simulink model "gm_parallel_prediction_and_cost_function_6phase"  (R2022a)
settings: Solver=FixedStepDiscrete  StartTime=0.0  StopTime=10.0  RelTol=1e-3
undefined symbols (not defined in the file or in its folder): f_c, L_d, L_q, L_x, L_y, p, psi_pm, R_ph
libraries: hdlmdlgenlib x338
(part 10 of 12)

== system gm_parallel_prediction_and_cost_function_6phase/Prediction_and_cost_function/Subsystem/MATLAB Function14/multiplier9 ==
  In1 : Inport
  In2 : Inport  Port=2
  multiplier9 : Product  Inputs=**  OutDataTypeStr=single  SampleTime=1e-08
  multiplier9_pd1 : Delay  DelayLength=6
  Out1 : Outport
  wires:
  multiplier9_pd1/1 -> Out1/1
  multiplier9/1 -> multiplier9_pd1/1
  In2/1 -> multiplier9/2
  In1/1 -> multiplier9/1

== system gm_parallel_prediction_and_cost_function_6phase/Prediction_and_cost_function/Subsystem/MATLAB Function14/square ==
  In1 : Inport
  In2 : Inport  Port=2
  square : Product  Inputs=**  OutDataTypeStr=single  SampleTime=1e-08
  square_pd1 : Delay  DelayLength=6
  Out1 : Outport
  wires:
  square_pd1/1 -> Out1/1
  square/1 -> square_pd1/1
  In2/1 -> square/2
  In1/1 -> square/1

== system gm_parallel_prediction_and_cost_function_6phase/Prediction_and_cost_function/Subsystem/MATLAB Function14/square1 ==
  In1 : Inport
  In2 : Inport  Port=2
  square1 : Product  Inputs=**  OutDataTypeStr=single  SampleTime=1e-08
  square1_pd1 : Delay  DelayLength=6
  Out1 : Outport
  wires:
  square1_pd1/1 -> Out1/1
  square1/1 -> square1_pd1/1
  In2/1 -> square1/2
  In1/1 -> square1/1

== system gm_parallel_prediction_and_cost_function_6phase/Prediction_and_cost_function/Subsystem/MATLAB Function14/square2 ==
  In1 : Inport
  In2 : Inport  Port=2
  square2 : Product  Inputs=**  OutDataTypeStr=single  SampleTime=1e-08
  square2_pd1 : Delay  DelayLength=6
  Out1 : Outport
  wires:
  square2_pd1/1 -> Out1/1
  square2/1 -> square2_pd1/1
  In2/1 -> square2/2
  In1/1 -> square2/1

== system gm_parallel_prediction_and_cost_function_6phase/Prediction_and_cost_function/Subsystem/MATLAB Function14/square3 ==
  In1 : Inport
  In2 : Inport  Port=2
  square3 : Product  Inputs=**  OutDataTypeStr=single  SampleTime=1e-08
  square3_pd1 : Delay  DelayLength=6
  Out1 : Outport
  wires:
  square3_pd1/1 -> Out1/1
  square3/1 -> square3_pd1/1
  In2/1 -> square3/2
  In1/1 -> square3/1

== system gm_parallel_prediction_and_cost_function_6phase/Prediction_and_cost_function/Subsystem/MATLAB Function14/subtract ==
  In1 : Inport
  In2 : Inport  Port=2
  subtract : Sum  Inputs=+-  OutDataTypeStr=single  SampleTime=1e-08
  subtract_pd1 : Delay  DelayLength=6
  Out1 : Outport
  wires:
  subtract_pd1/1 -> Out1/1
  subtract/1 -> subtract_pd1/1
  In2/1 -> subtract/2
  In1/1 -> subtract/1

== system gm_parallel_prediction_and_cost_function_6phase/Prediction_and_cost_function/Subsystem/MATLAB Function14/subtract1 ==
  In1 : Inport
  In2 : Inport  Port=2
  subtract1 : Sum  Inputs=+-  OutDataTypeStr=single  SampleTime=1e-08
  subtract1_pd1 : Delay  DelayLength=6
  Out1 : Outport
  wires:
  subtract1_pd1/1 -> Out1/1
  subtract1/1 -> subtract1_pd1/1
  In2/1 -> subtract1/2
  In1/1 -> subtract1/1

== system gm_parallel_prediction_and_cost_function_6phase/Prediction_and_cost_function/Subsystem/MATLAB Function14/subtract2 ==
  In1 : Inport
  In2 : Inport  Port=2
  subtract2 : Sum  Inputs=+-  OutDataTypeStr=single  SampleTime=1e-08
  subtract2_pd1 : Delay  DelayLength=6
  Out1 : Outport
  wires:
  subtract2_pd1/1 -> Out1/1
  subtract2/1 -> subtract2_pd1/1
  In2/1 -> subtract2/2
  In1/1 -> subtract2/1

== system gm_parallel_prediction_and_cost_function_6phase/Prediction_and_cost_function/Subsystem/MATLAB Function14/subtract3 ==
  In1 : Inport
  In2 : Inport  Port=2
  subtract3 : Sum  Inputs=+-  OutDataTypeStr=single  SampleTime=1e-08
  subtract3_pd1 : Delay  DelayLength=6
  Out1 : Outport
  wires:
  subtract3_pd1/1 -> Out1/1
  subtract3/1 -> subtract3_pd1/1
  In2/1 -> subtract3/2
  In1/1 -> subtract3/1

== system gm_parallel_prediction_and_cost_function_6phase/Prediction_and_cost_function/Subsystem/MATLAB Function14/subtract4 ==
  In1 : Inport
  In2 : Inport  Port=2
  subtract4 : Sum  Inputs=+-  OutDataTypeStr=single  SampleTime=1e-08
  subtract4_pd1 : Delay  DelayLength=6
  Out1 : Outport
  wires:
  subtract4_pd1/1 -> Out1/1
  subtract4/1 -> subtract4_pd1/1
  In2/1 -> subtract4/2
  In1/1 -> subtract4/1

== system gm_parallel_prediction_and_cost_function_6phase/Prediction_and_cost_function/Subsystem/MATLAB Function14/subtract5 ==
  In1 : Inport
  In2 : Inport  Port=2
  subtract5 : Sum  Inputs=+-  OutDataTypeStr=single  SampleTime=1e-08
  subtract5_pd1 : Delay  DelayLength=6
  Out1 : Outport
  wires:
  subtract5_pd1/1 -> Out1/1
  subtract5/1 -> subtract5_pd1/1
  In2/1 -> subtract5/2
  In1/1 -> subtract5/1

== system gm_parallel_prediction_and_cost_function_6phase/Prediction_and_cost_function/Subsystem/MATLAB Function14/subtract6 ==
  In1 : Inport
  In2 : Inport  Port=2
  subtract6 : Sum  Inputs=+-  OutDataTypeStr=single  SampleTime=1e-08
  subtract6_pd1 : Delay  DelayLength=6
  Out1 : Outport
  wires:
  subtract6_pd1/1 -> Out1/1
  subtract6/1 -> subtract6_pd1/1
  In2/1 -> subtract6/2
  In1/1 -> subtract6/1

== system gm_parallel_prediction_and_cost_function_6phase/Prediction_and_cost_function/Subsystem/MATLAB Function14/subtract7 ==
  In1 : Inport
  In2 : Inport  Port=2
  subtract7 : Sum  Inputs=+-  OutDataTypeStr=single  SampleTime=1e-08
  subtract7_pd1 : Delay  DelayLength=6
  Out1 : Outport
  wires:
  subtract7_pd1/1 -> Out1/1
  subtract7/1 -> subtract7_pd1/1
  In2/1 -> subtract7/2
  In1/1 -> subtract7/1

== system gm_parallel_prediction_and_cost_function_6phase/Prediction_and_cost_function/Subsystem/MATLAB Function14/subtract8 ==
  In1 : Inport
  In2 : Inport  Port=2
  subtract8 : Sum  Inputs=+-  OutDataTypeStr=single  SampleTime=1e-08
  subtract8_pd1 : Delay  DelayLength=6
  Out1 : Outport
  wires:
  subtract8_pd1/1 -> Out1/1
  subtract8/1 -> subtract8_pd1/1
  In2/1 -> subtract8/2
  In1/1 -> subtract8/1

== system gm_parallel_prediction_and_cost_function_6phase/Prediction_and_cost_function/Subsystem/MATLAB Function15/adder ==
  In1 : Inport
  In2 : Inport  Port=2
  adder : Sum  OutDataTypeStr=single  SampleTime=1e-08
  adder_pd1 : Delay  DelayLength=6
  Out1 : Outport
  wires:
  adder_pd1/1 -> Out1/1
  adder/1 -> adder_pd1/1
  In2/1 -> adder/2
  In1/1 -> adder/1

== system gm_parallel_prediction_and_cost_function_6phase/Prediction_and_cost_function/Subsystem/MATLAB Function15/adder1 ==
  In1 : Inport
  In2 : Inport  Port=2
  adder1 : Sum  OutDataTypeStr=single  SampleTime=1e-08
  adder1_pd1 : Delay  DelayLength=6
  Out1 : Outport
  wires:
  adder1_pd1/1 -> Out1/1
  adder1/1 -> adder1_pd1/1
  In2/1 -> adder1/2
  In1/1 -> adder1/1

== system gm_parallel_prediction_and_cost_function_6phase/Prediction_and_cost_function/Subsystem/MATLAB Function15/adder2 ==
  In1 : Inport
  In2 : Inport  Port=2
  adder2 : Sum  OutDataTypeStr=single  SampleTime=1e-08
  adder2_pd1 : Delay  DelayLength=6
  Out1 : Outport
  wires:
  adder2_pd1/1 -> Out1/1
  adder2/1 -> adder2_pd1/1
  In2/1 -> adder2/2
  In1/1 -> adder2/1

== system gm_parallel_prediction_and_cost_function_6phase/Prediction_and_cost_function/Subsystem/MATLAB Function15/adder3 ==
  In1 : Inport
  In2 : Inport  Port=2
  adder3 : Sum  OutDataTypeStr=single  SampleTime=1e-08
  adder3_pd1 : Delay  DelayLength=6
  Out1 : Outport
  wires:
  adder3_pd1/1 -> Out1/1
  adder3/1 -> adder3_pd1/1
  In2/1 -> adder3/2
  In1/1 -> adder3/1

== system gm_parallel_prediction_and_cost_function_6phase/Prediction_and_cost_function/Subsystem/MATLAB Function15/adder4 ==
  In1 : Inport
  In2 : Inport  Port=2
  adder4 : Sum  OutDataTypeStr=single  SampleTime=1e-08
  adder4_pd1 : Delay  DelayLength=6
  Out1 : Outport
  wires:
  adder4_pd1/1 -> Out1/1
  adder4/1 -> adder4_pd1/1
  In2/1 -> adder4/2
  In1/1 -> adder4/1

== system gm_parallel_prediction_and_cost_function_6phase/Prediction_and_cost_function/Subsystem/MATLAB Function15/adder5 ==
  In1 : Inport
  In2 : Inport  Port=2
  adder5 : Sum  OutDataTypeStr=single  SampleTime=1e-08
  adder5_pd1 : Delay  DelayLength=6
  Out1 : Outport
  wires:
  adder5_pd1/1 -> Out1/1
  adder5/1 -> adder5_pd1/1
  In2/1 -> adder5/2
  In1/1 -> adder5/1

== system gm_parallel_prediction_and_cost_function_6phase/Prediction_and_cost_function/Subsystem/MATLAB Function15/adder6 ==
  In1 : Inport
  In2 : Inport  Port=2
  adder6 : Sum  OutDataTypeStr=single  SampleTime=1e-08
  adder6_pd1 : Delay  DelayLength=6
  Out1 : Outport
  wires:
  adder6_pd1/1 -> Out1/1
  adder6/1 -> adder6_pd1/1
  In2/1 -> adder6/2
  In1/1 -> adder6/1

== system gm_parallel_prediction_and_cost_function_6phase/Prediction_and_cost_function/Subsystem/MATLAB Function15/adder7 ==
  In1 : Inport
  In2 : Inport  Port=2
  adder7 : Sum  OutDataTypeStr=single  SampleTime=1e-08
  adder7_pd1 : Delay  DelayLength=6
  Out1 : Outport
  wires:
  adder7_pd1/1 -> Out1/1
  adder7/1 -> adder7_pd1/1
  In2/1 -> adder7/2
  In1/1 -> adder7/1

== system gm_parallel_prediction_and_cost_function_6phase/Prediction_and_cost_function/Subsystem/MATLAB Function15/adder8 ==
  In1 : Inport
  In2 : Inport  Port=2
  adder8 : Sum  OutDataTypeStr=single  SampleTime=1e-08
  adder8_pd1 : Delay  DelayLength=6
  Out1 : Outport
  wires:
  adder8_pd1/1 -> Out1/1
  adder8/1 -> adder8_pd1/1
  In2/1 -> adder8/2
  In1/1 -> adder8/1

== system gm_parallel_prediction_and_cost_function_6phase/Prediction_and_cost_function/Subsystem/MATLAB Function15/multiplier ==
  In1 : Inport
  In2 : Inport  Port=2
  multiplier : Product  Inputs=**  OutDataTypeStr=single  SampleTime=1e-08
  multiplier_pd1 : Delay  DelayLength=6
  Out1 : Outport
  wires:
  multiplier_pd1/1 -> Out1/1
  multiplier/1 -> multiplier_pd1/1
  In2/1 -> multiplier/2
  In1/1 -> multiplier/1

== system gm_parallel_prediction_and_cost_function_6phase/Prediction_and_cost_function/Subsystem/MATLAB Function15/multiplier1 ==
  In1 : Inport
  In2 : Inport  Port=2
  multiplier1 : Product  Inputs=**  OutDataTypeStr=single  SampleTime=1e-08
  multiplier1_pd1 : Delay  DelayLength=6
  Out1 : Outport
  wires:
  multiplier1_pd1/1 -> Out1/1
  multiplier1/1 -> multiplier1_pd1/1
  In2/1 -> multiplier1/2
  In1/1 -> multiplier1/1

== system gm_parallel_prediction_and_cost_function_6phase/Prediction_and_cost_function/Subsystem/MATLAB Function15/multiplier10 ==
  In1 : Inport
  In2 : Inport  Port=2
  multiplier10 : Product  Inputs=**  OutDataTypeStr=single  SampleTime=1e-08
  multiplier10_pd1 : Delay  DelayLength=6
  Out1 : Outport
  wires:
  multiplier10_pd1/1 -> Out1/1
  multiplier10/1 -> multiplier10_pd1/1
  In2/1 -> multiplier10/2
  In1/1 -> multiplier10/1

== system gm_parallel_prediction_and_cost_function_6phase/Prediction_and_cost_function/Subsystem/MATLAB Function15/multiplier11 ==
  In1 : Inport
  In2 : Inport  Port=2
  multiplier11 : Product  Inputs=**  OutDataTypeStr=single  SampleTime=1e-08
  multiplier11_pd1 : Delay  DelayLength=6
  Out1 : Outport
  wires:
  multiplier11_pd1/1 -> Out1/1
  multiplier11/1 -> multiplier11_pd1/1
  In2/1 -> multiplier11/2
  In1/1 -> multiplier11/1

== system gm_parallel_prediction_and_cost_function_6phase/Prediction_and_cost_function/Subsystem/MATLAB Function15/multiplier2 ==
  In1 : Inport
  In2 : Inport  Port=2
  multiplier2 : Product  Inputs=**  OutDataTypeStr=single  SampleTime=1e-08
  multiplier2_pd1 : Delay  DelayLength=6
  Out1 : Outport
  wires:
  multiplier2_pd1/1 -> Out1/1
  multiplier2/1 -> multiplier2_pd1/1
  In2/1 -> multiplier2/2
  In1/1 -> multiplier2/1

== system gm_parallel_prediction_and_cost_function_6phase/Prediction_and_cost_function/Subsystem/MATLAB Function15/multiplier3 ==
  In1 : Inport
  In2 : Inport  Port=2
  multiplier3 : Product  Inputs=**  OutDataTypeStr=single  SampleTime=1e-08
  multiplier3_pd1 : Delay  DelayLength=6
  Out1 : Outport
  wires:
  multiplier3_pd1/1 -> Out1/1
  multiplier3/1 -> multiplier3_pd1/1
  In2/1 -> multiplier3/2
  In1/1 -> multiplier3/1

== system gm_parallel_prediction_and_cost_function_6phase/Prediction_and_cost_function/Subsystem/MATLAB Function15/multiplier4 ==
  In1 : Inport
  In2 : Inport  Port=2
  multiplier4 : Product  Inputs=**  OutDataTypeStr=single  SampleTime=1e-08
  multiplier4_pd1 : Delay  DelayLength=6
  Out1 : Outport
  wires:
  multiplier4_pd1/1 -> Out1/1
  multiplier4/1 -> multiplier4_pd1/1
  In2/1 -> multiplier4/2
  In1/1 -> multiplier4/1

== system gm_parallel_prediction_and_cost_function_6phase/Prediction_and_cost_function/Subsystem/MATLAB Function15/multiplier5 ==
  In1 : Inport
  In2 : Inport  Port=2
  multiplier5 : Product  Inputs=**  OutDataTypeStr=single  SampleTime=1e-08
  multiplier5_pd1 : Delay  DelayLength=6
  Out1 : Outport
  wires:
  multiplier5_pd1/1 -> Out1/1
  multiplier5/1 -> multiplier5_pd1/1
  In2/1 -> multiplier5/2
  In1/1 -> multiplier5/1

== system gm_parallel_prediction_and_cost_function_6phase/Prediction_and_cost_function/Subsystem/MATLAB Function15/multiplier6 ==
  In1 : Inport
  In2 : Inport  Port=2
  multiplier6 : Product  Inputs=**  OutDataTypeStr=single  SampleTime=1e-08
  multiplier6_pd1 : Delay  DelayLength=6
  Out1 : Outport
  wires:
  multiplier6_pd1/1 -> Out1/1
  multiplier6/1 -> multiplier6_pd1/1
  In2/1 -> multiplier6/2
  In1/1 -> multiplier6/1

== system gm_parallel_prediction_and_cost_function_6phase/Prediction_and_cost_function/Subsystem/MATLAB Function15/multiplier7 ==
  In1 : Inport
  In2 : Inport  Port=2
  multiplier7 : Product  Inputs=**  OutDataTypeStr=single  SampleTime=1e-08
  multiplier7_pd1 : Delay  DelayLength=6
  Out1 : Outport
  wires:
  multiplier7_pd1/1 -> Out1/1
  multiplier7/1 -> multiplier7_pd1/1
  In2/1 -> multiplier7/2
  In1/1 -> multiplier7/1

== system gm_parallel_prediction_and_cost_function_6phase/Prediction_and_cost_function/Subsystem/MATLAB Function15/multiplier8 ==
  In1 : Inport
  In2 : Inport  Port=2
  multiplier8 : Product  Inputs=**  OutDataTypeStr=single  SampleTime=1e-08
  multiplier8_pd1 : Delay  DelayLength=6
  Out1 : Outport
  wires:
  multiplier8_pd1/1 -> Out1/1
  multiplier8/1 -> multiplier8_pd1/1
  In2/1 -> multiplier8/2
  In1/1 -> multiplier8/1

== system gm_parallel_prediction_and_cost_function_6phase/Prediction_and_cost_function/Subsystem/MATLAB Function15/multiplier9 ==
  In1 : Inport
  In2 : Inport  Port=2
  multiplier9 : Product  Inputs=**  OutDataTypeStr=single  SampleTime=1e-08
  multiplier9_pd1 : Delay  DelayLength=6
  Out1 : Outport
  wires:
  multiplier9_pd1/1 -> Out1/1
  multiplier9/1 -> multiplier9_pd1/1
  In2/1 -> multiplier9/2
  In1/1 -> multiplier9/1

== system gm_parallel_prediction_and_cost_function_6phase/Prediction_and_cost_function/Subsystem/MATLAB Function15/square ==
  In1 : Inport
  In2 : Inport  Port=2
  square : Product  Inputs=**  OutDataTypeStr=single  SampleTime=1e-08
  square_pd1 : Delay  DelayLength=6
  Out1 : Outport
  wires:
  square_pd1/1 -> Out1/1
  square/1 -> square_pd1/1
  In2/1 -> square/2
  In1/1 -> square/1

== system gm_parallel_prediction_and_cost_function_6phase/Prediction_and_cost_function/Subsystem/MATLAB Function15/square1 ==
  In1 : Inport
  In2 : Inport  Port=2
  square1 : Product  Inputs=**  OutDataTypeStr=single  SampleTime=1e-08
  square1_pd1 : Delay  DelayLength=6
  Out1 : Outport
  wires:
  square1_pd1/1 -> Out1/1
  square1/1 -> square1_pd1/1
  In2/1 -> square1/2
  In1/1 -> square1/1

== system gm_parallel_prediction_and_cost_function_6phase/Prediction_and_cost_function/Subsystem/MATLAB Function15/square2 ==
  In1 : Inport
  In2 : Inport  Port=2
  square2 : Product  Inputs=**  OutDataTypeStr=single  SampleTime=1e-08
  square2_pd1 : Delay  DelayLength=6
  Out1 : Outport
  wires:
  square2_pd1/1 -> Out1/1
  square2/1 -> square2_pd1/1
  In2/1 -> square2/2
  In1/1 -> square2/1

== system gm_parallel_prediction_and_cost_function_6phase/Prediction_and_cost_function/Subsystem/MATLAB Function15/square3 ==
  In1 : Inport
  In2 : Inport  Port=2
  square3 : Product  Inputs=**  OutDataTypeStr=single  SampleTime=1e-08
  square3_pd1 : Delay  DelayLength=6
  Out1 : Outport
  wires:
  square3_pd1/1 -> Out1/1
  square3/1 -> square3_pd1/1
  In2/1 -> square3/2
  In1/1 -> square3/1

== system gm_parallel_prediction_and_cost_function_6phase/Prediction_and_cost_function/Subsystem/MATLAB Function15/subtract ==
  In1 : Inport
  In2 : Inport  Port=2
  subtract : Sum  Inputs=+-  OutDataTypeStr=single  SampleTime=1e-08
  subtract_pd1 : Delay  DelayLength=6
  Out1 : Outport
  wires:
  subtract_pd1/1 -> Out1/1
  subtract/1 -> subtract_pd1/1
  In2/1 -> subtract/2
  In1/1 -> subtract/1

== system gm_parallel_prediction_and_cost_function_6phase/Prediction_and_cost_function/Subsystem/MATLAB Function15/subtract1 ==
  In1 : Inport
  In2 : Inport  Port=2
  subtract1 : Sum  Inputs=+-  OutDataTypeStr=single  SampleTime=1e-08
  subtract1_pd1 : Delay  DelayLength=6
  Out1 : Outport
  wires:
  subtract1_pd1/1 -> Out1/1
  subtract1/1 -> subtract1_pd1/1
  In2/1 -> subtract1/2
  In1/1 -> subtract1/1

== system gm_parallel_prediction_and_cost_function_6phase/Prediction_and_cost_function/Subsystem/MATLAB Function15/subtract2 ==
  In1 : Inport
  In2 : Inport  Port=2
  subtract2 : Sum  Inputs=+-  OutDataTypeStr=single  SampleTime=1e-08
  subtract2_pd1 : Delay  DelayLength=6
  Out1 : Outport
  wires:
  subtract2_pd1/1 -> Out1/1
  subtract2/1 -> subtract2_pd1/1
  In2/1 -> subtract2/2
  In1/1 -> subtract2/1

== system gm_parallel_prediction_and_cost_function_6phase/Prediction_and_cost_function/Subsystem/MATLAB Function15/subtract3 ==
  In1 : Inport
  In2 : Inport  Port=2
  subtract3 : Sum  Inputs=+-  OutDataTypeStr=single  SampleTime=1e-08
  subtract3_pd1 : Delay  DelayLength=6
  Out1 : Outport
  wires:
  subtract3_pd1/1 -> Out1/1
  subtract3/1 -> subtract3_pd1/1
  In2/1 -> subtract3/2
  In1/1 -> subtract3/1

== system gm_parallel_prediction_and_cost_function_6phase/Prediction_and_cost_function/Subsystem/MATLAB Function15/subtract4 ==
  In1 : Inport
  In2 : Inport  Port=2
  subtract4 : Sum  Inputs=+-  OutDataTypeStr=single  SampleTime=1e-08
  subtract4_pd1 : Delay  DelayLength=6
  Out1 : Outport
  wires:
  subtract4_pd1/1 -> Out1/1
  subtract4/1 -> subtract4_pd1/1
  In2/1 -> subtract4/2
  In1/1 -> subtract4/1

== system gm_parallel_prediction_and_cost_function_6phase/Prediction_and_cost_function/Subsystem/MATLAB Function15/subtract5 ==
  In1 : Inport
  In2 : Inport  Port=2
  subtract5 : Sum  Inputs=+-  OutDataTypeStr=single  SampleTime=1e-08
  subtract5_pd1 : Delay  DelayLength=6
  Out1 : Outport
  wires:
  subtract5_pd1/1 -> Out1/1
  subtract5/1 -> subtract5_pd1/1
  In2/1 -> subtract5/2
  In1/1 -> subtract5/1

== system gm_parallel_prediction_and_cost_function_6phase/Prediction_and_cost_function/Subsystem/MATLAB Function15/subtract6 ==
  In1 : Inport
  In2 : Inport  Port=2
  subtract6 : Sum  Inputs=+-  OutDataTypeStr=single  SampleTime=1e-08
  subtract6_pd1 : Delay  DelayLength=6
  Out1 : Outport
  wires:
  subtract6_pd1/1 -> Out1/1
  subtract6/1 -> subtract6_pd1/1
  In2/1 -> subtract6/2
  In1/1 -> subtract6/1

== system gm_parallel_prediction_and_cost_function_6phase/Prediction_and_cost_function/Subsystem/MATLAB Function15/subtract7 ==
  In1 : Inport
  In2 : Inport  Port=2
  subtract7 : Sum  Inputs=+-  OutDataTypeStr=single  SampleTime=1e-08
  subtract7_pd1 : Delay  DelayLength=6
  Out1 : Outport
  wires:
  subtract7_pd1/1 -> Out1/1
  subtract7/1 -> subtract7_pd1/1
  In2/1 -> subtract7/2
  In1/1 -> subtract7/1

== system gm_parallel_prediction_and_cost_function_6phase/Prediction_and_cost_function/Subsystem/MATLAB Function15/subtract8 ==
  In1 : Inport
  In2 : Inport  Port=2
  subtract8 : Sum  Inputs=+-  OutDataTypeStr=single  SampleTime=1e-08
  subtract8_pd1 : Delay  DelayLength=6
  Out1 : Outport
  wires:
  subtract8_pd1/1 -> Out1/1
  subtract8/1 -> subtract8_pd1/1
  In2/1 -> subtract8/2
  In1/1 -> subtract8/1

== system gm_parallel_prediction_and_cost_function_6phase/Prediction_and_cost_function/Subsystem/MATLAB Function2/adder ==
  In1 : Inport
  In2 : Inport  Port=2
  adder : Sum  OutDataTypeStr=single  SampleTime=1e-08
  adder_pd1 : Delay  DelayLength=6
  Out1 : Outport
  wires:
  adder_pd1/1 -> Out1/1
  adder/1 -> adder_pd1/1
  In2/1 -> adder/2
  In1/1 -> adder/1

== system gm_parallel_prediction_and_cost_function_6phase/Prediction_and_cost_function/Subsystem/MATLAB Function2/adder1 ==
  In1 : Inport
  In2 : Inport  Port=2
  adder1 : Sum  OutDataTypeStr=single  SampleTime=1e-08
  adder1_pd1 : Delay  DelayLength=6
  Out1 : Outport
  wires:
  adder1_pd1/1 -> Out1/1
  adder1/1 -> adder1_pd1/1
  In2/1 -> adder1/2
  In1/1 -> adder1/1

== system gm_parallel_prediction_and_cost_function_6phase/Prediction_and_cost_function/Subsystem/MATLAB Function2/adder2 ==
  In1 : Inport
  In2 : Inport  Port=2
  adder2 : Sum  OutDataTypeStr=single  SampleTime=1e-08
  adder2_pd1 : Delay  DelayLength=6
  Out1 : Outport
  wires:
  adder2_pd1/1 -> Out1/1
  adder2/1 -> adder2_pd1/1
  In2/1 -> adder2/2
  In1/1 -> adder2/1

== system gm_parallel_prediction_and_cost_function_6phase/Prediction_and_cost_function/Subsystem/MATLAB Function2/adder3 ==
  In1 : Inport
  In2 : Inport  Port=2
  adder3 : Sum  OutDataTypeStr=single  SampleTime=1e-08
  adder3_pd1 : Delay  DelayLength=6
  Out1 : Outport
  wires:
  adder3_pd1/1 -> Out1/1
  adder3/1 -> adder3_pd1/1
  In2/1 -> adder3/2
  In1/1 -> adder3/1

== system gm_parallel_prediction_and_cost_function_6phase/Prediction_and_cost_function/Subsystem/MATLAB Function2/adder4 ==
  In1 : Inport
  In2 : Inport  Port=2
  adder4 : Sum  OutDataTypeStr=single  SampleTime=1e-08
  adder4_pd1 : Delay  DelayLength=6
  Out1 : Outport
  wires:
  adder4_pd1/1 -> Out1/1
  adder4/1 -> adder4_pd1/1
  In2/1 -> adder4/2
  In1/1 -> adder4/1

== system gm_parallel_prediction_and_cost_function_6phase/Prediction_and_cost_function/Subsystem/MATLAB Function2/adder5 ==
  In1 : Inport
  In2 : Inport  Port=2
  adder5 : Sum  OutDataTypeStr=single  SampleTime=1e-08
  adder5_pd1 : Delay  DelayLength=6
  Out1 : Outport
  wires:
  adder5_pd1/1 -> Out1/1
  adder5/1 -> adder5_pd1/1
  In2/1 -> adder5/2
  In1/1 -> adder5/1

== system gm_parallel_prediction_and_cost_function_6phase/Prediction_and_cost_function/Subsystem/MATLAB Function2/adder6 ==
  In1 : Inport
  In2 : Inport  Port=2
  adder6 : Sum  OutDataTypeStr=single  SampleTime=1e-08
  adder6_pd1 : Delay  DelayLength=6
  Out1 : Outport
  wires:
  adder6_pd1/1 -> Out1/1
  adder6/1 -> adder6_pd1/1
  In2/1 -> adder6/2
  In1/1 -> adder6/1

== system gm_parallel_prediction_and_cost_function_6phase/Prediction_and_cost_function/Subsystem/MATLAB Function2/adder7 ==
  In1 : Inport
  In2 : Inport  Port=2
  adder7 : Sum  OutDataTypeStr=single  SampleTime=1e-08
  adder7_pd1 : Delay  DelayLength=6
  Out1 : Outport
  wires:
  adder7_pd1/1 -> Out1/1
  adder7/1 -> adder7_pd1/1
  In2/1 -> adder7/2
  In1/1 -> adder7/1

== system gm_parallel_prediction_and_cost_function_6phase/Prediction_and_cost_function/Subsystem/MATLAB Function2/adder8 ==
  In1 : Inport
  In2 : Inport  Port=2
  adder8 : Sum  OutDataTypeStr=single  SampleTime=1e-08
  adder8_pd1 : Delay  DelayLength=6
  Out1 : Outport
  wires:
  adder8_pd1/1 -> Out1/1
  adder8/1 -> adder8_pd1/1
  In2/1 -> adder8/2
  In1/1 -> adder8/1

== system gm_parallel_prediction_and_cost_function_6phase/Prediction_and_cost_function/Subsystem/MATLAB Function2/multiplier ==
  In1 : Inport
  In2 : Inport  Port=2
  multiplier : Product  Inputs=**  OutDataTypeStr=single  SampleTime=1e-08
  multiplier_pd1 : Delay  DelayLength=6
  Out1 : Outport
  wires:
  multiplier_pd1/1 -> Out1/1
  multiplier/1 -> multiplier_pd1/1
  In2/1 -> multiplier/2
  In1/1 -> multiplier/1

== system gm_parallel_prediction_and_cost_function_6phase/Prediction_and_cost_function/Subsystem/MATLAB Function2/multiplier1 ==
  In1 : Inport
  In2 : Inport  Port=2
  multiplier1 : Product  Inputs=**  OutDataTypeStr=single  SampleTime=1e-08
  multiplier1_pd1 : Delay  DelayLength=6
  Out1 : Outport
  wires:
  multiplier1_pd1/1 -> Out1/1
  multiplier1/1 -> multiplier1_pd1/1
  In2/1 -> multiplier1/2
  In1/1 -> multiplier1/1

== system gm_parallel_prediction_and_cost_function_6phase/Prediction_and_cost_function/Subsystem/MATLAB Function2/multiplier10 ==
  In1 : Inport
  In2 : Inport  Port=2
  multiplier10 : Product  Inputs=**  OutDataTypeStr=single  SampleTime=1e-08
  multiplier10_pd1 : Delay  DelayLength=6
  Out1 : Outport
  wires:
  multiplier10_pd1/1 -> Out1/1
  multiplier10/1 -> multiplier10_pd1/1
  In2/1 -> multiplier10/2
  In1/1 -> multiplier10/1

== system gm_parallel_prediction_and_cost_function_6phase/Prediction_and_cost_function/Subsystem/MATLAB Function2/multiplier11 ==
  In1 : Inport
  In2 : Inport  Port=2
  multiplier11 : Product  Inputs=**  OutDataTypeStr=single  SampleTime=1e-08
  multiplier11_pd1 : Delay  DelayLength=6
  Out1 : Outport
  wires:
  multiplier11_pd1/1 -> Out1/1
  multiplier11/1 -> multiplier11_pd1/1
  In2/1 -> multiplier11/2
  In1/1 -> multiplier11/1

== system gm_parallel_prediction_and_cost_function_6phase/Prediction_and_cost_function/Subsystem/MATLAB Function2/multiplier2 ==
  In1 : Inport
  In2 : Inport  Port=2
  multiplier2 : Product  Inputs=**  OutDataTypeStr=single  SampleTime=1e-08
  multiplier2_pd1 : Delay  DelayLength=6
  Out1 : Outport
  wires:
  multiplier2_pd1/1 -> Out1/1
  multiplier2/1 -> multiplier2_pd1/1
  In2/1 -> multiplier2/2
  In1/1 -> multiplier2/1

== system gm_parallel_prediction_and_cost_function_6phase/Prediction_and_cost_function/Subsystem/MATLAB Function2/multiplier3 ==
  In1 : Inport
  In2 : Inport  Port=2
  multiplier3 : Product  Inputs=**  OutDataTypeStr=single  SampleTime=1e-08
  multiplier3_pd1 : Delay  DelayLength=6
  Out1 : Outport
  wires:
  multiplier3_pd1/1 -> Out1/1
  multiplier3/1 -> multiplier3_pd1/1
  In2/1 -> multiplier3/2
  In1/1 -> multiplier3/1

== system gm_parallel_prediction_and_cost_function_6phase/Prediction_and_cost_function/Subsystem/MATLAB Function2/multiplier4 ==
  In1 : Inport
  In2 : Inport  Port=2
  multiplier4 : Product  Inputs=**  OutDataTypeStr=single  SampleTime=1e-08
  multiplier4_pd1 : Delay  DelayLength=6
  Out1 : Outport
  wires:
  multiplier4_pd1/1 -> Out1/1
  multiplier4/1 -> multiplier4_pd1/1
  In2/1 -> multiplier4/2
  In1/1 -> multiplier4/1

== system gm_parallel_prediction_and_cost_function_6phase/Prediction_and_cost_function/Subsystem/MATLAB Function2/multiplier5 ==
  In1 : Inport
  In2 : Inport  Port=2
  multiplier5 : Product  Inputs=**  OutDataTypeStr=single  SampleTime=1e-08
  multiplier5_pd1 : Delay  DelayLength=6
  Out1 : Outport
  wires:
  multiplier5_pd1/1 -> Out1/1
  multiplier5/1 -> multiplier5_pd1/1
  In2/1 -> multiplier5/2
  In1/1 -> multiplier5/1

== system gm_parallel_prediction_and_cost_function_6phase/Prediction_and_cost_function/Subsystem/MATLAB Function2/multiplier6 ==
  In1 : Inport
  In2 : Inport  Port=2
  multiplier6 : Product  Inputs=**  OutDataTypeStr=single  SampleTime=1e-08
  multiplier6_pd1 : Delay  DelayLength=6
  Out1 : Outport
  wires:
  multiplier6_pd1/1 -> Out1/1
  multiplier6/1 -> multiplier6_pd1/1
  In2/1 -> multiplier6/2
  In1/1 -> multiplier6/1

== system gm_parallel_prediction_and_cost_function_6phase/Prediction_and_cost_function/Subsystem/MATLAB Function2/multiplier7 ==
  In1 : Inport
  In2 : Inport  Port=2
  multiplier7 : Product  Inputs=**  OutDataTypeStr=single  SampleTime=1e-08
  multiplier7_pd1 : Delay  DelayLength=6
  Out1 : Outport
  wires:
  multiplier7_pd1/1 -> Out1/1
  multiplier7/1 -> multiplier7_pd1/1
  In2/1 -> multiplier7/2
  In1/1 -> multiplier7/1

== system gm_parallel_prediction_and_cost_function_6phase/Prediction_and_cost_function/Subsystem/MATLAB Function2/multiplier8 ==
  In1 : Inport
  In2 : Inport  Port=2
  multiplier8 : Product  Inputs=**  OutDataTypeStr=single  SampleTime=1e-08
  multiplier8_pd1 : Delay  DelayLength=6
  Out1 : Outport
  wires:
  multiplier8_pd1/1 -> Out1/1
  multiplier8/1 -> multiplier8_pd1/1
  In2/1 -> multiplier8/2
  In1/1 -> multiplier8/1

== system gm_parallel_prediction_and_cost_function_6phase/Prediction_and_cost_function/Subsystem/MATLAB Function2/multiplier9 ==
  In1 : Inport
  In2 : Inport  Port=2
  multiplier9 : Product  Inputs=**  OutDataTypeStr=single  SampleTime=1e-08
  multiplier9_pd1 : Delay  DelayLength=6
  Out1 : Outport
  wires:
  multiplier9_pd1/1 -> Out1/1
  multiplier9/1 -> multiplier9_pd1/1
  In2/1 -> multiplier9/2
  In1/1 -> multiplier9/1

== system gm_parallel_prediction_and_cost_function_6phase/Prediction_and_cost_function/Subsystem/MATLAB Function2/square ==
  In1 : Inport
  In2 : Inport  Port=2
  square : Product  Inputs=**  OutDataTypeStr=single  SampleTime=1e-08
  square_pd1 : Delay  DelayLength=6
  Out1 : Outport
  wires:
  square_pd1/1 -> Out1/1
  square/1 -> square_pd1/1
  In2/1 -> square/2
  In1/1 -> square/1

== system gm_parallel_prediction_and_cost_function_6phase/Prediction_and_cost_function/Subsystem/MATLAB Function2/square1 ==
  In1 : Inport
  In2 : Inport  Port=2
  square1 : Product  Inputs=**  OutDataTypeStr=single  SampleTime=1e-08
  square1_pd1 : Delay  DelayLength=6
  Out1 : Outport
  wires:
  square1_pd1/1 -> Out1/1
  square1/1 -> square1_pd1/1
  In2/1 -> square1/2
  In1/1 -> square1/1

== system gm_parallel_prediction_and_cost_function_6phase/Prediction_and_cost_function/Subsystem/MATLAB Function2/square2 ==
  In1 : Inport
  In2 : Inport  Port=2
  square2 : Product  Inputs=**  OutDataTypeStr=single  SampleTime=1e-08
  square2_pd1 : Delay  DelayLength=6
  Out1 : Outport
  wires:
  square2_pd1/1 -> Out1/1
  square2/1 -> square2_pd1/1
  In2/1 -> square2/2
  In1/1 -> square2/1

== system gm_parallel_prediction_and_cost_function_6phase/Prediction_and_cost_function/Subsystem/MATLAB Function2/square3 ==
  In1 : Inport
  In2 : Inport  Port=2
  square3 : Product  Inputs=**  OutDataTypeStr=single  SampleTime=1e-08
  square3_pd1 : Delay  DelayLength=6
  Out1 : Outport
  wires:
  square3_pd1/1 -> Out1/1
  square3/1 -> square3_pd1/1
  In2/1 -> square3/2
  In1/1 -> square3/1

== system gm_parallel_prediction_and_cost_function_6phase/Prediction_and_cost_function/Subsystem/MATLAB Function2/subtract ==
  In1 : Inport
  In2 : Inport  Port=2
  subtract : Sum  Inputs=+-  OutDataTypeStr=single  SampleTime=1e-08
  subtract_pd1 : Delay  DelayLength=6
  Out1 : Outport
  wires:
  subtract_pd1/1 -> Out1/1
  subtract/1 -> subtract_pd1/1
  In2/1 -> subtract/2
  In1/1 -> subtract/1

== system gm_parallel_prediction_and_cost_function_6phase/Prediction_and_cost_function/Subsystem/MATLAB Function2/subtract1 ==
  In1 : Inport
  In2 : Inport  Port=2
  subtract1 : Sum  Inputs=+-  OutDataTypeStr=single  SampleTime=1e-08
  subtract1_pd1 : Delay  DelayLength=6
  Out1 : Outport
  wires:
  subtract1_pd1/1 -> Out1/1
  subtract1/1 -> subtract1_pd1/1
  In2/1 -> subtract1/2
  In1/1 -> subtract1/1

== system gm_parallel_prediction_and_cost_function_6phase/Prediction_and_cost_function/Subsystem/MATLAB Function2/subtract2 ==
  In1 : Inport
  In2 : Inport  Port=2
  subtract2 : Sum  Inputs=+-  OutDataTypeStr=single  SampleTime=1e-08
  subtract2_pd1 : Delay  DelayLength=6
  Out1 : Outport
  wires:
  subtract2_pd1/1 -> Out1/1
  subtract2/1 -> subtract2_pd1/1
  In2/1 -> subtract2/2
  In1/1 -> subtract2/1

== system gm_parallel_prediction_and_cost_function_6phase/Prediction_and_cost_function/Subsystem/MATLAB Function2/subtract3 ==
  In1 : Inport
  In2 : Inport  Port=2
  subtract3 : Sum  Inputs=+-  OutDataTypeStr=single  SampleTime=1e-08
  subtract3_pd1 : Delay  DelayLength=6
  Out1 : Outport
  wires:
  subtract3_pd1/1 -> Out1/1
  subtract3/1 -> subtract3_pd1/1
  In2/1 -> subtract3/2
  In1/1 -> subtract3/1

== system gm_parallel_prediction_and_cost_function_6phase/Prediction_and_cost_function/Subsystem/MATLAB Function2/subtract4 ==
  In1 : Inport
  In2 : Inport  Port=2
  subtract4 : Sum  Inputs=+-  OutDataTypeStr=single  SampleTime=1e-08
  subtract4_pd1 : Delay  DelayLength=6
  Out1 : Outport
  wires:
  subtract4_pd1/1 -> Out1/1
  subtract4/1 -> subtract4_pd1/1
  In2/1 -> subtract4/2
  In1/1 -> subtract4/1

== system gm_parallel_prediction_and_cost_function_6phase/Prediction_and_cost_function/Subsystem/MATLAB Function2/subtract5 ==
  In1 : Inport
  In2 : Inport  Port=2
  subtract5 : Sum  Inputs=+-  OutDataTypeStr=single  SampleTime=1e-08
  subtract5_pd1 : Delay  DelayLength=6
  Out1 : Outport
  wires:
  subtract5_pd1/1 -> Out1/1
  subtract5/1 -> subtract5_pd1/1
  In2/1 -> subtract5/2
  In1/1 -> subtract5/1

== system gm_parallel_prediction_and_cost_function_6phase/Prediction_and_cost_function/Subsystem/MATLAB Function2/subtract6 ==
  In1 : Inport
  In2 : Inport  Port=2
  subtract6 : Sum  Inputs=+-  OutDataTypeStr=single  SampleTime=1e-08
  subtract6_pd1 : Delay  DelayLength=6
  Out1 : Outport
  wires:
  subtract6_pd1/1 -> Out1/1
  subtract6/1 -> subtract6_pd1/1
  In2/1 -> subtract6/2
  In1/1 -> subtract6/1

== system gm_parallel_prediction_and_cost_function_6phase/Prediction_and_cost_function/Subsystem/MATLAB Function2/subtract7 ==
  In1 : Inport
  In2 : Inport  Port=2
  subtract7 : Sum  Inputs=+-  OutDataTypeStr=single  SampleTime=1e-08
  subtract7_pd1 : Delay  DelayLength=6
  Out1 : Outport
  wires:
  subtract7_pd1/1 -> Out1/1
  subtract7/1 -> subtract7_pd1/1
  In2/1 -> subtract7/2
  In1/1 -> subtract7/1

== system gm_parallel_prediction_and_cost_function_6phase/Prediction_and_cost_function/Subsystem/MATLAB Function2/subtract8 ==
  In1 : Inport
  In2 : Inport  Port=2
  subtract8 : Sum  Inputs=+-  OutDataTypeStr=single  SampleTime=1e-08
  subtract8_pd1 : Delay  DelayLength=6
  Out1 : Outport
  wires:
  subtract8_pd1/1 -> Out1/1
  subtract8/1 -> subtract8_pd1/1
  In2/1 -> subtract8/2
  In1/1 -> subtract8/1

== system gm_parallel_prediction_and_cost_function_6phase/Prediction_and_cost_function/Subsystem/MATLAB Function3/adder ==
  In1 : Inport
  In2 : Inport  Port=2
  adder : Sum  OutDataTypeStr=single  SampleTime=1e-08
  adder_pd1 : Delay  DelayLength=6
  Out1 : Outport
  wires:
  adder_pd1/1 -> Out1/1
  adder/1 -> adder_pd1/1
  In2/1 -> adder/2
  In1/1 -> adder/1

== system gm_parallel_prediction_and_cost_function_6phase/Prediction_and_cost_function/Subsystem/MATLAB Function3/adder1 ==
  In1 : Inport
  In2 : Inport  Port=2
  adder1 : Sum  OutDataTypeStr=single  SampleTime=1e-08
  adder1_pd1 : Delay  DelayLength=6
  Out1 : Outport
  wires:
  adder1_pd1/1 -> Out1/1
  adder1/1 -> adder1_pd1/1
  In2/1 -> adder1/2
  In1/1 -> adder1/1

== system gm_parallel_prediction_and_cost_function_6phase/Prediction_and_cost_function/Subsystem/MATLAB Function3/adder2 ==
  In1 : Inport
  In2 : Inport  Port=2
  adder2 : Sum  OutDataTypeStr=single  SampleTime=1e-08
  adder2_pd1 : Delay  DelayLength=6
  Out1 : Outport
  wires:
  adder2_pd1/1 -> Out1/1
  adder2/1 -> adder2_pd1/1
  In2/1 -> adder2/2
  In1/1 -> adder2/1

== system gm_parallel_prediction_and_cost_function_6phase/Prediction_and_cost_function/Subsystem/MATLAB Function3/adder3 ==
  In1 : Inport
  In2 : Inport  Port=2
  adder3 : Sum  OutDataTypeStr=single  SampleTime=1e-08
  adder3_pd1 : Delay  DelayLength=6
  Out1 : Outport
  wires:
  adder3_pd1/1 -> Out1/1
  adder3/1 -> adder3_pd1/1
  In2/1 -> adder3/2
  In1/1 -> adder3/1

== system gm_parallel_prediction_and_cost_function_6phase/Prediction_and_cost_function/Subsystem/MATLAB Function3/adder4 ==
  In1 : Inport
  In2 : Inport  Port=2
  adder4 : Sum  OutDataTypeStr=single  SampleTime=1e-08
  adder4_pd1 : Delay  DelayLength=6
  Out1 : Outport
  wires:
  adder4_pd1/1 -> Out1/1
  adder4/1 -> adder4_pd1/1
  In2/1 -> adder4/2
  In1/1 -> adder4/1

== system gm_parallel_prediction_and_cost_function_6phase/Prediction_and_cost_function/Subsystem/MATLAB Function3/adder5 ==
  In1 : Inport
  In2 : Inport  Port=2
  adder5 : Sum  OutDataTypeStr=single  SampleTime=1e-08
  adder5_pd1 : Delay  DelayLength=6
  Out1 : Outport
  wires:
  adder5_pd1/1 -> Out1/1
  adder5/1 -> adder5_pd1/1
  In2/1 -> adder5/2
  In1/1 -> adder5/1

== system gm_parallel_prediction_and_cost_function_6phase/Prediction_and_cost_function/Subsystem/MATLAB Function3/adder6 ==
  In1 : Inport
  In2 : Inport  Port=2
  adder6 : Sum  OutDataTypeStr=single  SampleTime=1e-08
  adder6_pd1 : Delay  DelayLength=6
  Out1 : Outport
  wires:
  adder6_pd1/1 -> Out1/1
  adder6/1 -> adder6_pd1/1
  In2/1 -> adder6/2
  In1/1 -> adder6/1

== system gm_parallel_prediction_and_cost_function_6phase/Prediction_and_cost_function/Subsystem/MATLAB Function3/adder7 ==
  In1 : Inport
  In2 : Inport  Port=2
  adder7 : Sum  OutDataTypeStr=single  SampleTime=1e-08
  adder7_pd1 : Delay  DelayLength=6
  Out1 : Outport
  wires:
  adder7_pd1/1 -> Out1/1
  adder7/1 -> adder7_pd1/1
  In2/1 -> adder7/2
  In1/1 -> adder7/1

== system gm_parallel_prediction_and_cost_function_6phase/Prediction_and_cost_function/Subsystem/MATLAB Function3/adder8 ==
  In1 : Inport
  In2 : Inport  Port=2
  adder8 : Sum  OutDataTypeStr=single  SampleTime=1e-08
  adder8_pd1 : Delay  DelayLength=6
  Out1 : Outport
  wires:
  adder8_pd1/1 -> Out1/1
  adder8/1 -> adder8_pd1/1
  In2/1 -> adder8/2
  In1/1 -> adder8/1

== system gm_parallel_prediction_and_cost_function_6phase/Prediction_and_cost_function/Subsystem/MATLAB Function3/multiplier ==
  In1 : Inport
  In2 : Inport  Port=2
  multiplier : Product  Inputs=**  OutDataTypeStr=single  SampleTime=1e-08
  multiplier_pd1 : Delay  DelayLength=6
  Out1 : Outport
  wires:
  multiplier_pd1/1 -> Out1/1
  multiplier/1 -> multiplier_pd1/1
  In2/1 -> multiplier/2
  In1/1 -> multiplier/1

== system gm_parallel_prediction_and_cost_function_6phase/Prediction_and_cost_function/Subsystem/MATLAB Function3/multiplier1 ==
  In1 : Inport
  In2 : Inport  Port=2
  multiplier1 : Product  Inputs=**  OutDataTypeStr=single  SampleTime=1e-08
  multiplier1_pd1 : Delay  DelayLength=6
  Out1 : Outport
  wires:
  multiplier1_pd1/1 -> Out1/1
  multiplier1/1 -> multiplier1_pd1/1
  In2/1 -> multiplier1/2
  In1/1 -> multiplier1/1

== system gm_parallel_prediction_and_cost_function_6phase/Prediction_and_cost_function/Subsystem/MATLAB Function3/multiplier10 ==
  In1 : Inport
  In2 : Inport  Port=2
  multiplier10 : Product  Inputs=**  OutDataTypeStr=single  SampleTime=1e-08
  multiplier10_pd1 : Delay  DelayLength=6
  Out1 : Outport
  wires:
  multiplier10_pd1/1 -> Out1/1
  multiplier10/1 -> multiplier10_pd1/1
  In2/1 -> multiplier10/2
  In1/1 -> multiplier10/1

== system gm_parallel_prediction_and_cost_function_6phase/Prediction_and_cost_function/Subsystem/MATLAB Function3/multiplier11 ==
  In1 : Inport
  In2 : Inport  Port=2
  multiplier11 : Product  Inputs=**  OutDataTypeStr=single  SampleTime=1e-08
  multiplier11_pd1 : Delay  DelayLength=6
  Out1 : Outport
  wires:
  multiplier11_pd1/1 -> Out1/1
  multiplier11/1 -> multiplier11_pd1/1
  In2/1 -> multiplier11/2
  In1/1 -> multiplier11/1

== system gm_parallel_prediction_and_cost_function_6phase/Prediction_and_cost_function/Subsystem/MATLAB Function3/multiplier2 ==
  In1 : Inport
  In2 : Inport  Port=2
  multiplier2 : Product  Inputs=**  OutDataTypeStr=single  SampleTime=1e-08
  multiplier2_pd1 : Delay  DelayLength=6
  Out1 : Outport
  wires:
  multiplier2_pd1/1 -> Out1/1
  multiplier2/1 -> multiplier2_pd1/1
  In2/1 -> multiplier2/2
  In1/1 -> multiplier2/1

== system gm_parallel_prediction_and_cost_function_6phase/Prediction_and_cost_function/Subsystem/MATLAB Function3/multiplier3 ==
  In1 : Inport
  In2 : Inport  Port=2
  multiplier3 : Product  Inputs=**  OutDataTypeStr=single  SampleTime=1e-08
  multiplier3_pd1 : Delay  DelayLength=6
  Out1 : Outport
  wires:
  multiplier3_pd1/1 -> Out1/1
  multiplier3/1 -> multiplier3_pd1/1
  In2/1 -> multiplier3/2
  In1/1 -> multiplier3/1

== system gm_parallel_prediction_and_cost_function_6phase/Prediction_and_cost_function/Subsystem/MATLAB Function3/multiplier4 ==
  In1 : Inport
  In2 : Inport  Port=2
  multiplier4 : Product  Inputs=**  OutDataTypeStr=single  SampleTime=1e-08
  multiplier4_pd1 : Delay  DelayLength=6
  Out1 : Outport
  wires:
  multiplier4_pd1/1 -> Out1/1
  multiplier4/1 -> multiplier4_pd1/1
  In2/1 -> multiplier4/2
  In1/1 -> multiplier4/1

== system gm_parallel_prediction_and_cost_function_6phase/Prediction_and_cost_function/Subsystem/MATLAB Function3/multiplier5 ==
  In1 : Inport
  In2 : Inport  Port=2
  multiplier5 : Product  Inputs=**  OutDataTypeStr=single  SampleTime=1e-08
  multiplier5_pd1 : Delay  DelayLength=6
  Out1 : Outport
  wires:
  multiplier5_pd1/1 -> Out1/1
  multiplier5/1 -> multiplier5_pd1/1
  In2/1 -> multiplier5/2
  In1/1 -> multiplier5/1

== system gm_parallel_prediction_and_cost_function_6phase/Prediction_and_cost_function/Subsystem/MATLAB Function3/multiplier6 ==
  In1 : Inport
  In2 : Inport  Port=2
  multiplier6 : Product  Inputs=**  OutDataTypeStr=single  SampleTime=1e-08
  multiplier6_pd1 : Delay  DelayLength=6
  Out1 : Outport
  wires:
  multiplier6_pd1/1 -> Out1/1
  multiplier6/1 -> multiplier6_pd1/1
  In2/1 -> multiplier6/2
  In1/1 -> multiplier6/1

== system gm_parallel_prediction_and_cost_function_6phase/Prediction_and_cost_function/Subsystem/MATLAB Function3/multiplier7 ==
  In1 : Inport
  In2 : Inport  Port=2
  multiplier7 : Product  Inputs=**  OutDataTypeStr=single  SampleTime=1e-08
  multiplier7_pd1 : Delay  DelayLength=6
  Out1 : Outport
  wires:
  multiplier7_pd1/1 -> Out1/1
  multiplier7/1 -> multiplier7_pd1/1
  In2/1 -> multiplier7/2
  In1/1 -> multiplier7/1

== system gm_parallel_prediction_and_cost_function_6phase/Prediction_and_cost_function/Subsystem/MATLAB Function3/multiplier8 ==
  In1 : Inport
  In2 : Inport  Port=2
  multiplier8 : Product  Inputs=**  OutDataTypeStr=single  SampleTime=1e-08
  multiplier8_pd1 : Delay  DelayLength=6
  Out1 : Outport
  wires:
  multiplier8_pd1/1 -> Out1/1
  multiplier8/1 -> multiplier8_pd1/1
  In2/1 -> multiplier8/2
  In1/1 -> multiplier8/1

== system gm_parallel_prediction_and_cost_function_6phase/Prediction_and_cost_function/Subsystem/MATLAB Function3/multiplier9 ==
  In1 : Inport
  In2 : Inport  Port=2
  multiplier9 : Product  Inputs=**  OutDataTypeStr=single  SampleTime=1e-08
  multiplier9_pd1 : Delay  DelayLength=6
  Out1 : Outport
  wires:
  multiplier9_pd1/1 -> Out1/1
  multiplier9/1 -> multiplier9_pd1/1
  In2/1 -> multiplier9/2
  In1/1 -> multiplier9/1

== system gm_parallel_prediction_and_cost_function_6phase/Prediction_and_cost_function/Subsystem/MATLAB Function3/square ==
  In1 : Inport
  In2 : Inport  Port=2
  square : Product  Inputs=**  OutDataTypeStr=single  SampleTime=1e-08
  square_pd1 : Delay  DelayLength=6
  Out1 : Outport
  wires:
  square_pd1/1 -> Out1/1
  square/1 -> square_pd1/1
  In2/1 -> square/2
  In1/1 -> square/1

== system gm_parallel_prediction_and_cost_function_6phase/Prediction_and_cost_function/Subsystem/MATLAB Function3/square1 ==
  In1 : Inport
  In2 : Inport  Port=2
  square1 : Product  Inputs=**  OutDataTypeStr=single  SampleTime=1e-08
  square1_pd1 : Delay  DelayLength=6
  Out1 : Outport
  wires:
  square1_pd1/1 -> Out1/1
  square1/1 -> square1_pd1/1
  In2/1 -> square1/2
  In1/1 -> square1/1

== system gm_parallel_prediction_and_cost_function_6phase/Prediction_and_cost_function/Subsystem/MATLAB Function3/square2 ==
  In1 : Inport
  In2 : Inport  Port=2
  square2 : Product  Inputs=**  OutDataTypeStr=single  SampleTime=1e-08
  square2_pd1 : Delay  DelayLength=6
  Out1 : Outport
  wires:
  square2_pd1/1 -> Out1/1
  square2/1 -> square2_pd1/1
  In2/1 -> square2/2
  In1/1 -> square2/1

== system gm_parallel_prediction_and_cost_function_6phase/Prediction_and_cost_function/Subsystem/MATLAB Function3/square3 ==
  In1 : Inport
  In2 : Inport  Port=2
  square3 : Product  Inputs=**  OutDataTypeStr=single  SampleTime=1e-08
  square3_pd1 : Delay  DelayLength=6
  Out1 : Outport
  wires:
  square3_pd1/1 -> Out1/1
  square3/1 -> square3_pd1/1
  In2/1 -> square3/2
  In1/1 -> square3/1

== system gm_parallel_prediction_and_cost_function_6phase/Prediction_and_cost_function/Subsystem/MATLAB Function3/subtract ==
  In1 : Inport
  In2 : Inport  Port=2
  subtract : Sum  Inputs=+-  OutDataTypeStr=single  SampleTime=1e-08
  subtract_pd1 : Delay  DelayLength=6
  Out1 : Outport
  wires:
  subtract_pd1/1 -> Out1/1
  subtract/1 -> subtract_pd1/1
  In2/1 -> subtract/2
  In1/1 -> subtract/1

== system gm_parallel_prediction_and_cost_function_6phase/Prediction_and_cost_function/Subsystem/MATLAB Function3/subtract1 ==
  In1 : Inport
  In2 : Inport  Port=2
  subtract1 : Sum  Inputs=+-  OutDataTypeStr=single  SampleTime=1e-08
  subtract1_pd1 : Delay  DelayLength=6
  Out1 : Outport
  wires:
  subtract1_pd1/1 -> Out1/1
  subtract1/1 -> subtract1_pd1/1
  In2/1 -> subtract1/2
  In1/1 -> subtract1/1

== system gm_parallel_prediction_and_cost_function_6phase/Prediction_and_cost_function/Subsystem/MATLAB Function3/subtract2 ==
  In1 : Inport
  In2 : Inport  Port=2
  subtract2 : Sum  Inputs=+-  OutDataTypeStr=single  SampleTime=1e-08
  subtract2_pd1 : Delay  DelayLength=6
  Out1 : Outport
  wires:
  subtract2_pd1/1 -> Out1/1
  subtract2/1 -> subtract2_pd1/1
  In2/1 -> subtract2/2
  In1/1 -> subtract2/1

== system gm_parallel_prediction_and_cost_function_6phase/Prediction_and_cost_function/Subsystem/MATLAB Function3/subtract3 ==
  In1 : Inport
  In2 : Inport  Port=2
  subtract3 : Sum  Inputs=+-  OutDataTypeStr=single  SampleTime=1e-08
  subtract3_pd1 : Delay  DelayLength=6
  Out1 : Outport
  wires:
  subtract3_pd1/1 -> Out1/1
  subtract3/1 -> subtract3_pd1/1
  In2/1 -> subtract3/2
  In1/1 -> subtract3/1

== system gm_parallel_prediction_and_cost_function_6phase/Prediction_and_cost_function/Subsystem/MATLAB Function3/subtract4 ==
  In1 : Inport
  In2 : Inport  Port=2
  subtract4 : Sum  Inputs=+-  OutDataTypeStr=single  SampleTime=1e-08
  subtract4_pd1 : Delay  DelayLength=6
  Out1 : Outport
  wires:
  subtract4_pd1/1 -> Out1/1
  subtract4/1 -> subtract4_pd1/1
  In2/1 -> subtract4/2
  In1/1 -> subtract4/1

== system gm_parallel_prediction_and_cost_function_6phase/Prediction_and_cost_function/Subsystem/MATLAB Function3/subtract5 ==
  In1 : Inport
  In2 : Inport  Port=2
  subtract5 : Sum  Inputs=+-  OutDataTypeStr=single  SampleTime=1e-08
  subtract5_pd1 : Delay  DelayLength=6
  Out1 : Outport
  wires:
  subtract5_pd1/1 -> Out1/1
  subtract5/1 -> subtract5_pd1/1
  In2/1 -> subtract5/2
  In1/1 -> subtract5/1

== system gm_parallel_prediction_and_cost_function_6phase/Prediction_and_cost_function/Subsystem/MATLAB Function3/subtract6 ==
  In1 : Inport
  In2 : Inport  Port=2
  subtract6 : Sum  Inputs=+-  OutDataTypeStr=single  SampleTime=1e-08
  subtract6_pd1 : Delay  DelayLength=6
  Out1 : Outport
  wires:
  subtract6_pd1/1 -> Out1/1
  subtract6/1 -> subtract6_pd1/1
  In2/1 -> subtract6/2
  In1/1 -> subtract6/1

== system gm_parallel_prediction_and_cost_function_6phase/Prediction_and_cost_function/Subsystem/MATLAB Function3/subtract7 ==
  In1 : Inport
  In2 : Inport  Port=2
  subtract7 : Sum  Inputs=+-  OutDataTypeStr=single  SampleTime=1e-08
  subtract7_pd1 : Delay  DelayLength=6
  Out1 : Outport
  wires:
  subtract7_pd1/1 -> Out1/1
  subtract7/1 -> subtract7_pd1/1
  In2/1 -> subtract7/2
  In1/1 -> subtract7/1

== system gm_parallel_prediction_and_cost_function_6phase/Prediction_and_cost_function/Subsystem/MATLAB Function3/subtract8 ==
  In1 : Inport
  In2 : Inport  Port=2
  subtract8 : Sum  Inputs=+-  OutDataTypeStr=single  SampleTime=1e-08
  subtract8_pd1 : Delay  DelayLength=6
  Out1 : Outport
  wires:
  subtract8_pd1/1 -> Out1/1
  subtract8/1 -> subtract8_pd1/1
  In2/1 -> subtract8/2
  In1/1 -> subtract8/1

== system gm_parallel_prediction_and_cost_function_6phase/Prediction_and_cost_function/Subsystem/MATLAB Function4/adder ==
  In1 : Inport
  In2 : Inport  Port=2
  adder : Sum  OutDataTypeStr=single  SampleTime=1e-08
  adder_pd1 : Delay  DelayLength=6
  Out1 : Outport
  wires:
  adder_pd1/1 -> Out1/1
  adder/1 -> adder_pd1/1
  In2/1 -> adder/2
  In1/1 -> adder/1

== system gm_parallel_prediction_and_cost_function_6phase/Prediction_and_cost_function/Subsystem/MATLAB Function4/adder1 ==
  In1 : Inport
  In2 : Inport  Port=2
  adder1 : Sum  OutDataTypeStr=single  SampleTime=1e-08
  adder1_pd1 : Delay  DelayLength=6
  Out1 : Outport
  wires:
  adder1_pd1/1 -> Out1/1
  adder1/1 -> adder1_pd1/1
  In2/1 -> adder1/2
  In1/1 -> adder1/1

== system gm_parallel_prediction_and_cost_function_6phase/Prediction_and_cost_function/Subsystem/MATLAB Function4/adder2 ==
  In1 : Inport
  In2 : Inport  Port=2
  adder2 : Sum  OutDataTypeStr=single  SampleTime=1e-08
  adder2_pd1 : Delay  DelayLength=6
  Out1 : Outport
  wires:
  adder2_pd1/1 -> Out1/1
  adder2/1 -> adder2_pd1/1
  In2/1 -> adder2/2
  In1/1 -> adder2/1

== system gm_parallel_prediction_and_cost_function_6phase/Prediction_and_cost_function/Subsystem/MATLAB Function4/adder3 ==
  In1 : Inport
  In2 : Inport  Port=2
  adder3 : Sum  OutDataTypeStr=single  SampleTime=1e-08
  adder3_pd1 : Delay  DelayLength=6
  Out1 : Outport
  wires:
  adder3_pd1/1 -> Out1/1
  adder3/1 -> adder3_pd1/1
  In2/1 -> adder3/2
  In1/1 -> adder3/1

== system gm_parallel_prediction_and_cost_function_6phase/Prediction_and_cost_function/Subsystem/MATLAB Function4/adder4 ==
  In1 : Inport
  In2 : Inport  Port=2
  adder4 : Sum  OutDataTypeStr=single  SampleTime=1e-08
  adder4_pd1 : Delay  DelayLength=6
  Out1 : Outport
  wires:
  adder4_pd1/1 -> Out1/1
  adder4/1 -> adder4_pd1/1
  In2/1 -> adder4/2
  In1/1 -> adder4/1

== system gm_parallel_prediction_and_cost_function_6phase/Prediction_and_cost_function/Subsystem/MATLAB Function4/adder5 ==
  In1 : Inport
  In2 : Inport  Port=2
  adder5 : Sum  OutDataTypeStr=single  SampleTime=1e-08
  adder5_pd1 : Delay  DelayLength=6
  Out1 : Outport
  wires:
  adder5_pd1/1 -> Out1/1
  adder5/1 -> adder5_pd1/1
  In2/1 -> adder5/2
  In1/1 -> adder5/1

== system gm_parallel_prediction_and_cost_function_6phase/Prediction_and_cost_function/Subsystem/MATLAB Function4/adder6 ==
  In1 : Inport
  In2 : Inport  Port=2
  adder6 : Sum  OutDataTypeStr=single  SampleTime=1e-08
  adder6_pd1 : Delay  DelayLength=6
  Out1 : Outport
  wires:
  adder6_pd1/1 -> Out1/1
  adder6/1 -> adder6_pd1/1
  In2/1 -> adder6/2
  In1/1 -> adder6/1
